simulink model "CartPole"  (R2024a)
settings: Solver=VariableStepAuto  StartTime=0.0  StopTime=5  RelTol=1e-6
undefined symbols (not defined in the file): A, Acl, Appo, Atot, B, Bppo, Btot, C, Cppo, Ctot, D, Dppo, Dtot, g, l, M, m, Ts, x0
settings Model: Creator=Personal  LastModifiedBy=Personal

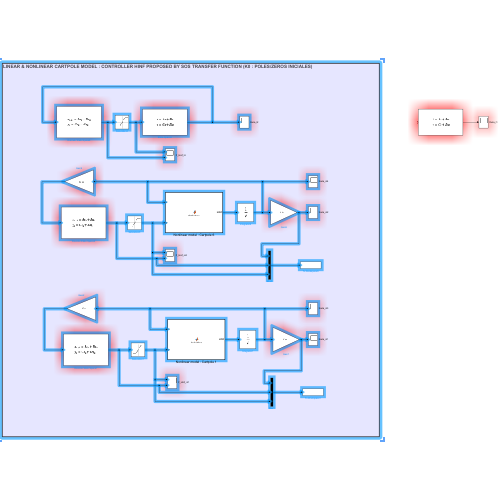
[thumbnail: Simulink's stored preview of the top-level diagram]
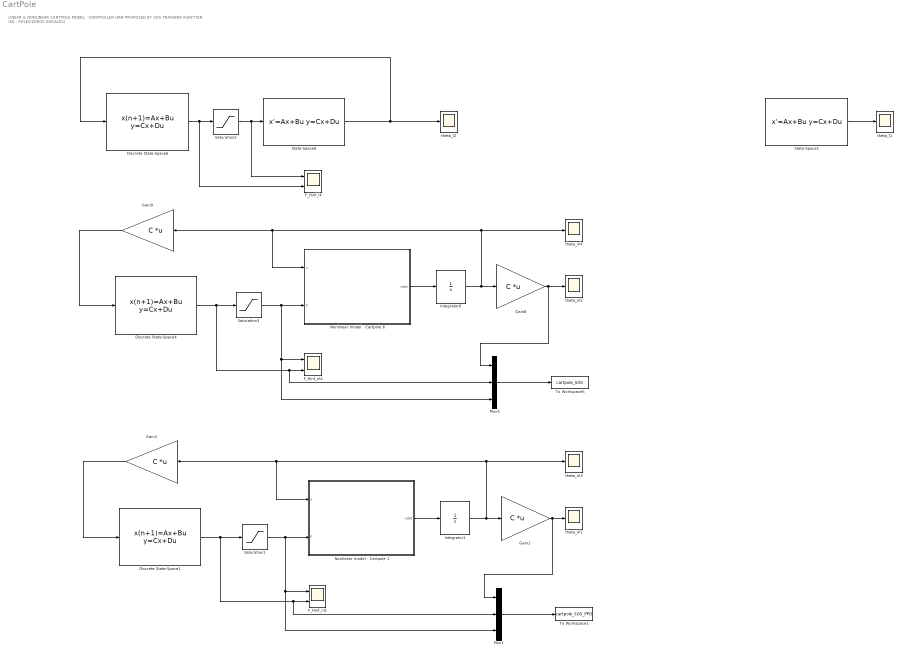
== system CartPole ==
  note: LINEAR & NONLINEAR CARTPOLE MODEL : CONTROLLER HINF PROPOSED BY SOS TRANSFER FUNCTION (K0 : POLES/ZEROS INICIALES)
  Discrete State-Space1 : DiscreteStateSpace  A=Appo  B=Bppo  C=Cppo  D=Dppo  InitialCondition=zeros(length(Appo),1)  SampleTime=Ts
  Discrete State-Space4 : DiscreteStateSpace  A=Atot  B=Btot  C=Ctot  D=Dtot  InitialCondition=zeros(length(Atot),1)  SampleTime=Ts
  Discrete State-Space6 : DiscreteStateSpace  A=Atot  B=Btot  C=Ctot  D=Dtot  InitialCondition=zeros(length(Atot),1)  SampleTime=Ts
  F_Hinf_l4 : Scope  NumInputPorts=2
  F_Hinf_nl1 : Scope  NumInputPorts=2
  F_Hinf_nl4 : Scope  NumInputPorts=2
  Gain{1..2,8..9} (4 alike) : Gain  Gain=C  Multiplication=Matrix(K*u)
  Integrator1 : Integrator  InitialCondition=x0
  Integrator6 : Integrator  InitialCondition=x0
  Mux1 : Mux  Inputs=3
  Mux5 : Mux  Inputs=3
  "Nonlinear model : Cartpole 1" : MATLAB Function  TreatAsAtomicUnit=on
  "Nonlinear model : Cartpole 6" : MATLAB Function  TreatAsAtomicUnit=on
  Saturation1 : Saturate  UpperLimit=15  LowerLimit=-15
  Saturation2 : Saturate  UpperLimit=15  LowerLimit=-15
  Saturation3 : Saturate  UpperLimit=15  LowerLimit=-15
  State-Space1 : StateSpace  A=Acl  B=zeros(length(Acl),1)  C=eye(4,length(Acl))  D=zeros(4,1)  InitialCondition=[x0;0;0;0;0]
  State-Space6 : StateSpace  A=A  B=B  C=C  D=D  InitialCondition=x0
  To Workspace1 : ToWorkspace  VariableName=cartpole_SOS_PPO  SaveFormat=Timeseries  SampleTime=-1
  To Workspace5 : ToWorkspace  VariableName=cartpole_SOS  SaveFormat=Timeseries  SampleTime=-1
  theta_l1 : Scope
  theta_l2 : Scope
  theta_nl{1..4} (4 alike) : Scope
  wires:
  Gain9/1 -> Discrete State-Space4/1
  Discrete State-Space4/1 -> Saturation3/1, F_Hinf_nl4/2, Mux5/2
  "Nonlinear model : Cartpole 6"/1(xdot) -> Integrator6/1
  Discrete State-Space6/1 -> Saturation2/1, F_Hinf_l4/2
  Gain8/1 -> Mux5/1, theta_nl2/1
  Integrator6/1 -> Gain8/1, theta_nl4/1, "Nonlinear model : Cartpole 6"/1(x), Gain9/1
  Mux5/1 -> To Workspace5/1
  Mux1/1 -> To Workspace1/1
  Integrator1/1 -> Gain1/1, theta_nl3/1, "Nonlinear model : Cartpole 1"/1(x), Gain2/1
  Saturation1/1 -> "Nonlinear model : Cartpole 1"/2(F), Mux1/3, F_Hinf_nl1/1
  Discrete State-Space1/1 -> F_Hinf_nl1/2, Mux1/2, Saturation1/1
  Gain1/1 -> Mux1/1, theta_nl1/1
  "Nonlinear model : Cartpole 1"/1(xdot) -> Integrator1/1
  Gain2/1 -> Discrete State-Space1/1
  State-Space6/1 -> Discrete State-Space6/1, theta_l2/1
  Saturation2/1 -> F_Hinf_l4/1, State-Space6/1
  State-Space1/1 -> theta_l1/1
  Saturation3/1 -> "Nonlinear model : Cartpole 6"/2(F), Mux5/3, F_Hinf_nl4/1

== matlab function CartPole/Nonlinear model : Cartpole 1 ==
  data: x input; xdot output; F input; M parameter; m parameter; g parameter; l parameter
function xdot = derivatives(x,F, M, m, g, l)
%xdot as state-variables vector (includes second and first order dynamics)
% x = [x, xdot, theta, thetadot]' (4,1)
%Initial conditions (IC) are given in ODE SOLVER (1/s). 
den = M + m -m*cos(x(3))^2;
xdot = zeros(4,1);
xdot(1) = x(2);
xdot(2) = (-m*g*x(3)*cos(x(3)) + m*l*x(4)^2*sin(x(3)))/den + (1/den)*F;
xdot(3) = x(4);
xdot(4) = ((M + m)*g*sin(x(3)) - cos(x(3))*m*l*x(4)^2*sin(x(3)))/(l*den) ...
    - (cos(x(3))/(l*den))*F;

== matlab function CartPole/Nonlinear model : Cartpole 6 ==
  data: x input; xdot output; F input; M parameter; m parameter; g parameter; l parameter
function xdot = derivatives(x,F, M, m, g, l)
%xdot as state-variables vector (includes second and first order dynamics)
% x = [x, xdot, theta, thetadot]' (4,1)
%Initial conditions (IC) are given in ODE SOLVER (1/s). 
den = M + m -m*cos(x(3))^2;
xdot = zeros(4,1);
xdot(1) = x(2);
xdot(2) = (-m*g*x(3)*cos(x(3)) + m*l*x(4)^2*sin(x(3)))/den + (1/den)*F;
xdot(3) = x(4);
xdot(4) = ((M + m)*g*sin(x(3)) - cos(x(3))*m*l*x(4)^2*sin(x(3)))/(l*den) ...
    - (cos(x(3))/(l*den))*F;
